simulink model "qsim"  (R2022b)
settings: Solver=VariableStepAuto  StartTime=0.0  StopTime=tmax  MaxStep=dt  RelTol=1e-3
values from neighbouring files (symbols this model uses):
  area = pi*0.42^2    (= 0.554176944093)    [black_brant_vc.m]
  burning_rate = mfuel/burn_time    (= 31.4003701419)    [black_brant_vc.m]
  Cd = [0.386 0.329 0.325 0.469 0.488 0.434 0.389 0.328 0.287 0.255 0.216      0.194 0.184 0.169 0.164 0.154 ]'    [questions.m]
  centrifugal_force = false    [questions.m]
  fthrust = 69.4*10^3    (= 69400)    [black_brant_vc.m]
  G = 6.67430*10^-11    (= 6.6743e-11)    [questions.m]
  M = [0.1 0.5 0.8 1 1.2 1.5 2 2.5 3 3.5 4      4.5 5 5.5 6 6.5]'    [questions.m]
  mfuel = 1018    [black_brant_vc.m]
  mpayload = 100    [black_brant_vc.m]
  mrocket = 243    [black_brant_vc.m]
  nozzle_area = pi*0.34^2    (= 0.363168110755)    [black_brant_vc.m]
  pitch = s*rad    [questions.m]
  v0x = sin(pitch)*v0    [questions.m]
  v0y = sin(pitch)*v0    [questions.m]
  Ve = Isp * G0    [black_brant_vc.m]
  veq = 0    [questions.m]
  x0 = 0    [questions.m]
  y0 = 0    [questions.m]
undefined symbols (not defined in the file or in its folder): D0, H, mearth, P0, r_earth
libraries: simulink x4
settings Model: Creator=mitch  LastModifiedBy=mitch
settings DataIOCC: ReturnWorkspaceOutputs=off

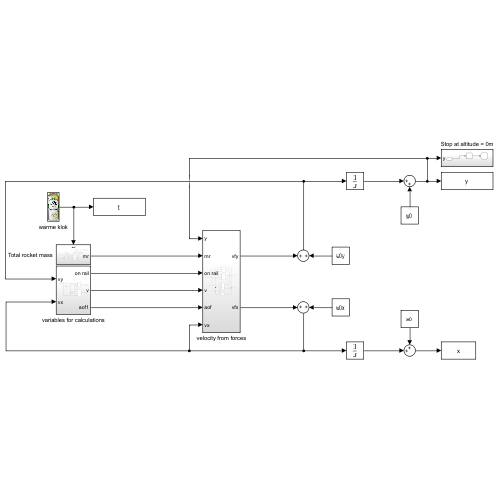
[thumbnail: Simulink's stored preview of the top-level diagram]
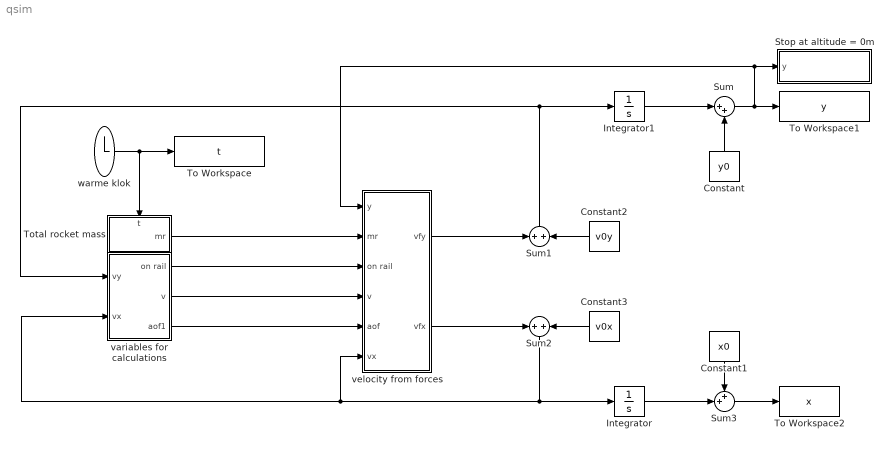
== system qsim ==
  Constant : Constant  Value=y0
  Constant1 : Constant  Value=x0
  Constant2 : Constant  Value=v0y
  Constant3 : Constant  Value=v0x
  Integrator : Integrator
  Integrator1 : Integrator
  Stop at altitude = 0m : Subsystem
  Sum : Sum  Inputs=|++
  Sum1 : Sum
  Sum2 : Sum
  Sum3 : Sum  Inputs=++|
  To Workspace : ToWorkspace  VariableName=t  SampleTime=-1
  To Workspace1 : ToWorkspace  VariableName=y  SampleTime=-1
  To Workspace2 : ToWorkspace  VariableName=x  SampleTime=-1
  Total rocket mass : Subsystem
      settings: PortSchema="{\"entries\":[{\"content\":{\"sides\":[{\"content\":{\"connectorIds\":[]},\"type\":\"ConnectorPlacement.EquallySpacedRectSide\",\"uuid\":\"93486deb-20ea-4256-be89-9e1e72dbb09d\"},{\"content\":{\"connectorIds\":[\"Out1\"],\"side\":\"RIGHT\"},\"type\":\"ConnectorPlacement.EquallySpacedRectSide\",\"uuid\":\"ed0e6263-0b76-41b6-b681-94567fbb2fbf\"},{\"content\":{\"connectorIds\":[\"In1\"],\"side\":\"TOP\"},\"type\":\"ConnectorPlacement.EquallySpacedRectSide\",\"uuid\":\"518b6907-16db-46e5-a33c-d197bc16f302\"}]},\"type\":\"ConnectorPlacement.EquallySpacedConnector\",\"uuid\":\"f80f25e1-82c3-4b04-8094-90952900617d\"}],\"packageUris\":[\"http://schema.mathworks.com/mf0/Connector/R2020b\"],\"version\":\"1.0\"}"
  variables for calculations : Subsystem
  velocity from forces : Subsystem
  warme klok : Clock
      mask Display: image(imread('klok.jpg'))
  wires:
  warme klok/1 -> To Workspace/1, Total rocket mass/1(t)
  Integrator1/1 -> Sum/1
  Sum/1 -> To Workspace1/1, Stop at altitude = 0m/1(y), velocity from forces/1(y)
  Constant/1 -> Sum/2
  Sum1/1 -> Integrator1/1, variables for calculations/1(vy)
  Integrator/1 -> Sum3/2
  Sum3/1 -> To Workspace2/1
  Constant1/1 -> Sum3/1
  Total rocket mass/1(mr) -> velocity from forces/2(mr)
  Sum2/1 -> Integrator/1, variables for calculations/2(vx), velocity from forces/6(vx)
  Constant3/1 -> Sum2/2
  velocity from forces/2(vfx) -> Sum2/1
  variables for calculations/1(on rail) -> velocity from forces/3(on rail)
  variables for calculations/2(v) -> velocity from forces/4(v)
  variables for calculations/3(aof1) -> velocity from forces/5(aof)
  velocity from forces/1(vfy) -> Sum1/1
  Constant2/1 -> Sum1/2

== system qsim/Stop at altitude = 0m ==
  y : Inport
  IsNegative : simulink/Logic and Bit Operations/Compare To Zero  relop=<  OutDataTypeStr=boolean
      settings: LibrarySourceBlock=|
      | simulink/Quick Insert/Logic and Bit
      | Operations/IsNegative
  Stop Simulation : Stop
  wires:
  IsNegative/1 -> Stop Simulation/1
  y/1 -> IsNegative/1

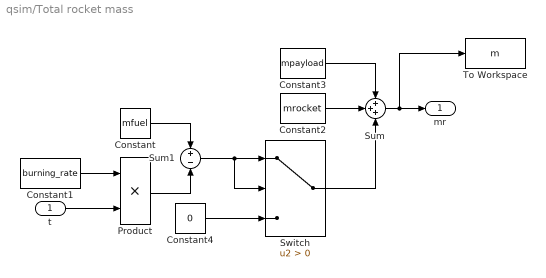
== system qsim/Total rocket mass ==
  t : Inport
  Constant : Constant  Value=mfuel
  Constant1 : Constant  Value=burning_rate
  Constant2 : Constant  Value=mrocket
  Constant3 : Constant  Value=mpayload
  Constant4 : Constant  Value=0
  Product : Product
  Sum : Sum  Inputs=+++
  Sum1 : Sum  Inputs=+-
  Switch : Switch  Criteria=u2 > Threshold  SaturateOnIntegerOverflow=off  InputSameDT=off
  To Workspace : ToWorkspace  VariableName=m  SampleTime=-1
  mr : Outport
  wires:
  Constant3/1 -> Sum/1
  Constant1/1 -> Product/1
  t/1 -> Product/2
  Constant2/1 -> Sum/2
  Constant4/1 -> Switch/3
  Constant/1 -> Sum1/1
  Sum1/1 -> Switch/1, Switch/2
  Product/1 -> Sum1/2
  Switch/1 -> Sum/3
  Sum/1 -> To Workspace/1, mr/1

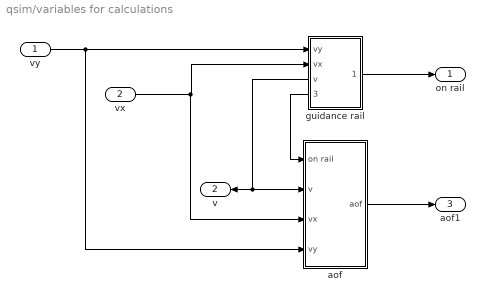
== system qsim/variables for calculations ==
  vy : Inport
  vx : Inport  Port=2
  aof : Subsystem
  guidance rail : Subsystem
      settings: PortSchema="{\"entries\":[{\"content\":{\"sides\":[{\"content\":{\"connectorIds\":[\"In1\",\"In2\",\"Out2\",\"Out3\"]},\"type\":\"ConnectorPlacement.EquallySpacedRectSide\",\"uuid\":\"58d90baa-7253-4a77-a7a7-25666266f078\"},{\"content\":{\"connectorIds\":[\"Out1\"],\"side\":\"RIGHT\"},\"type\":\"ConnectorPlacement.EquallySpacedRectSide\",\"uuid\":\"983a7505-aeb9-4571-80eb-2e5812b070ec\"},{\"content\":{\"connectorIds\":[],\"side\":\"TOP\"},\"type\":\"ConnectorPlacement.EquallySpacedRectSide\",\"uuid\":\"a1f35db6-1c46-42f7-bbcb-98ac4c623d07\"}]},\"type\":\"ConnectorPlacement.EquallySpacedConnector\",\"uuid\":\"73284847-f8fe-421a-b1ed-4d4b0b6e1462\"}],\"packageUris\":[\"http://schema.mathworks.com/mf0/Connector/R2020b\"],\"version\":\"1.0\"}"
  on rail : Outport
  v : Outport  Port=2
  aof1 : Outport  Port=3
  wires:
  guidance rail/3(on rail2) -> aof/1(on rail)
  guidance rail/1(on rail) -> on rail/1
  aof/1(aof) -> aof1/1
  vx/1 -> aof/3(vx), guidance rail/2(vx)
  guidance rail/2(v) -> v/1, aof/2(v)
  vy/1 -> aof/4(vy), guidance rail/1(vy)

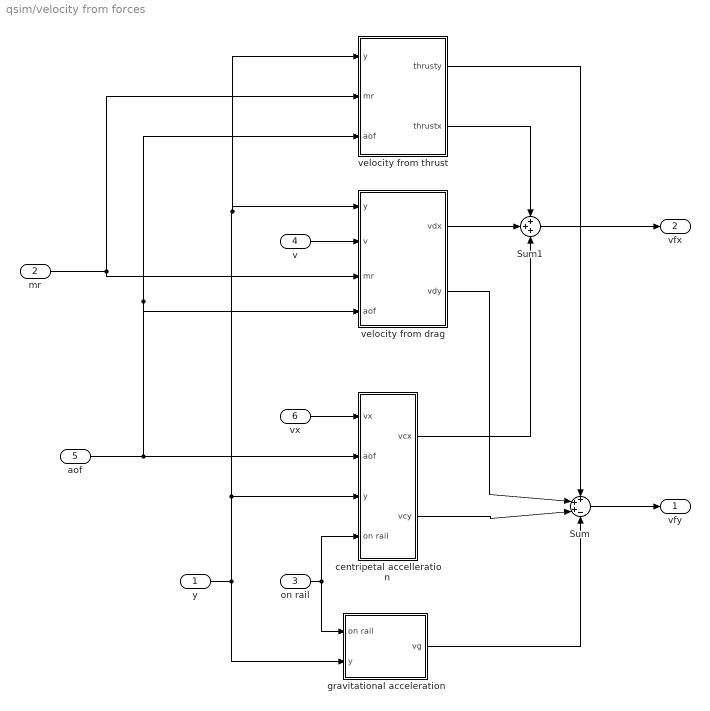
== system qsim/velocity from forces ==
  y : Inport
  mr : Inport  Port=2
  on rail : Inport  Port=3
  v : Inport  Port=4
  aof : Inport  Port=5
  vx : Inport  Port=6
  Sum : Sum  Inputs=+++-
  Sum1 : Sum  Inputs=+++
  centripetal accelleration : Subsystem
  gravitational acceleration : Subsystem
  velocity from drag : Subsystem
  velocity from thrust : Subsystem
  vfy : Outport
  vfx : Outport  Port=2
  wires:
  centripetal accelleration/2(vcy) -> Sum/3
  y/1 -> velocity from thrust/1(y), velocity from drag/1(y), centripetal accelleration/3(y), gravitational acceleration/2(y)
  on rail/1 -> centripetal accelleration/4(on rail), gravitational acceleration/1(on rail)
  mr/1 -> velocity from thrust/2(mr), velocity from drag/3(mr)
  velocity from drag/1(vdx) -> Sum1/2
  v/1 -> velocity from drag/2(v)
  gravitational acceleration/1(vg) -> Sum/4
  vx/1 -> centripetal accelleration/1(vx)
  centripetal accelleration/1(vcx) -> Sum1/3
  velocity from drag/2(vdy) -> Sum/2
  aof/1 -> centripetal accelleration/2(aof), velocity from drag/4(aof), velocity from thrust/3(aof)
  velocity from thrust/2(thrustx) -> Sum1/1
  velocity from thrust/1(thrusty) -> Sum/1
  Sum1/1 -> vfx/1
  Sum/1 -> vfy/1

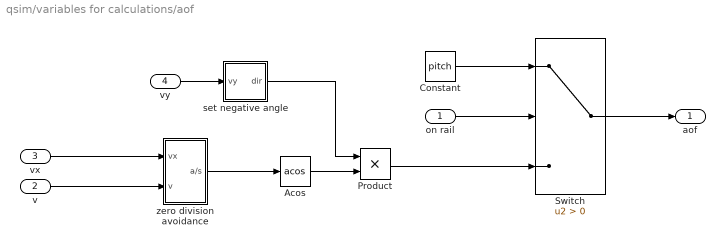
== system qsim/variables for calculations/aof ==
  on rail : Inport
  v : Inport  Port=2
  vx : Inport  Port=3
  vy : Inport  Port=4
  Acos : Trigonometry  Operator=acos
  Constant : Constant  Value=pitch
  Product : Product
  Switch : Switch  Criteria=u2 > Threshold  SaturateOnIntegerOverflow=off  InputSameDT=off
  set negative angle : Subsystem
  zero division avoidance : Subsystem
  aof : Outport
  wires:
  Switch/1 -> aof/1
  Constant/1 -> Switch/1
  on rail/1 -> Switch/2
  vx/1 -> zero division avoidance/1(vx)
  v/1 -> zero division avoidance/2(v)
  zero division avoidance/1(a/s) -> Acos/1
  Acos/1 -> Product/2
  Product/1 -> Switch/3
  vy/1 -> set negative angle/1(vy)
  set negative angle/1(dir) -> Product/1

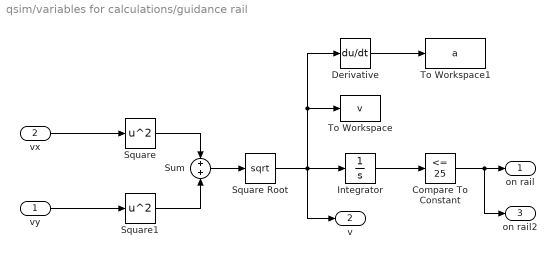
== system qsim/variables for calculations/guidance rail ==
  vy : Inport
  vx : Inport  Port=2
  Compare To Constant : simulink/Logic and Bit Operations/Compare To Constant  relop=<=  const=25  OutDataTypeStr=boolean
  Derivative : Derivative
  Integrator : Integrator
  Square : Math  Operator=square
  Square Root : Sqrt
  Square1 : Math  Operator=square
  Sum : Sum
  To Workspace : ToWorkspace  VariableName=v  SampleTime=-1
  To Workspace1 : ToWorkspace  VariableName=a  SampleTime=-1
  on rail : Outport
  v : Outport  Port=2
  on rail2 : Outport  Port=3
  wires:
  vy/1 -> Square1/1
  Square1/1 -> Sum/2
  Square/1 -> Sum/1
  Sum/1 -> Square Root/1
  Square Root/1 -> v/1, Derivative/1, To Workspace/1, Integrator/1
  Integrator/1 -> Compare To Constant/1
  Compare To Constant/1 -> on rail2/1, on rail/1
  vx/1 -> Square/1
  Derivative/1 -> To Workspace1/1

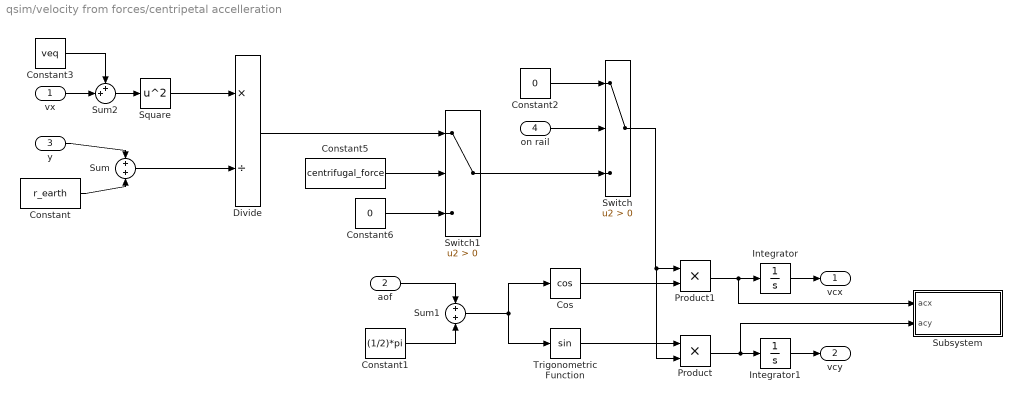
== system qsim/velocity from forces/centripetal accelleration ==
  vx : Inport
  aof : Inport  Port=2
  y : Inport  Port=3
  on rail : Inport  Port=4
  Constant : Constant  Value=r_earth
  Constant1 : Constant  Value=(1/2)*pi
  Constant2 : Constant  Value=0
  Constant3 : Constant  Value=veq
  Constant5 : Constant  Value=centrifugal_force
  Constant6 : Constant  Value=0
  Cos : Trigonometry  Operator=cos
  Divide : Product  Inputs=*/
  Integrator : Integrator
  Integrator1 : Integrator
  Product : Product
  Product1 : Product
  Square : Math  Operator=square
  Subsystem : Subsystem
  Sum : Sum
  Sum1 : Sum
  Sum2 : Sum  Inputs=++|
  Switch : Switch  Criteria=u2 > Threshold  SaturateOnIntegerOverflow=off  InputSameDT=off
  Switch1 : Switch  Criteria=u2 > Threshold  SaturateOnIntegerOverflow=off  InputSameDT=off
  Trigonometric Function : Trigonometry
  vcx : Outport
  vcy : Outport  Port=2
  wires:
  Constant/1 -> Sum/2
  y/1 -> Sum/1
  Square/1 -> Divide/1
  Sum/1 -> Divide/2
  aof/1 -> Sum1/1
  Constant1/1 -> Sum1/2
  Sum1/1 -> Trigonometric Function/1, Cos/1
  Cos/1 -> Product1/2
  Trigonometric Function/1 -> Product/1
  Integrator/1 -> vcx/1
  Product1/1 -> Subsystem/1(acx), Integrator/1
  Integrator1/1 -> vcy/1
  Product/1 -> Subsystem/2(acy), Integrator1/1
  Constant5/1 -> Switch1/2
  Constant6/1 -> Switch1/3
  Divide/1 -> Switch1/1
  on rail/1 -> Switch/2
  Constant2/1 -> Switch/1
  Switch1/1 -> Switch/3
  Switch/1 -> Product/2, Product1/1
  Sum2/1 -> Square/1
  vx/1 -> Sum2/2
  Constant3/1 -> Sum2/1

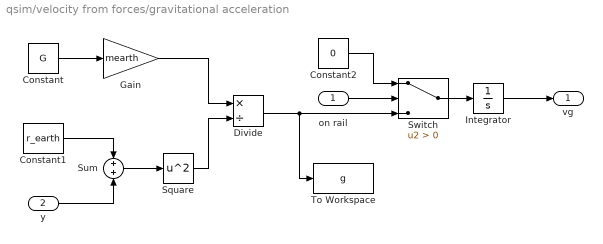
== system qsim/velocity from forces/gravitational acceleration ==
  on rail : Inport
  y : Inport  Port=2
  Constant : Constant  Value=G
  Constant1 : Constant  Value=r_earth
  Constant2 : Constant  Value=0
  Divide : Product  Inputs=*/
  Gain : Gain  Gain=mearth
  Integrator : Integrator
  Square : Math  Operator=square
  Sum : Sum
  Switch : Switch  Criteria=u2 > Threshold  SaturateOnIntegerOverflow=off  InputSameDT=off
  To Workspace : ToWorkspace  VariableName=g  SampleTime=-1
  vg : Outport
  wires:
  y/1 -> Sum/2
  Constant1/1 -> Sum/1
  Constant/1 -> Gain/1
  Gain/1 -> Divide/1
  Sum/1 -> Square/1
  Square/1 -> Divide/2
  Divide/1 -> Switch/3, To Workspace/1
  on rail/1 -> Switch/2
  Switch/1 -> Integrator/1
  Integrator/1 -> vg/1
  Constant2/1 -> Switch/1

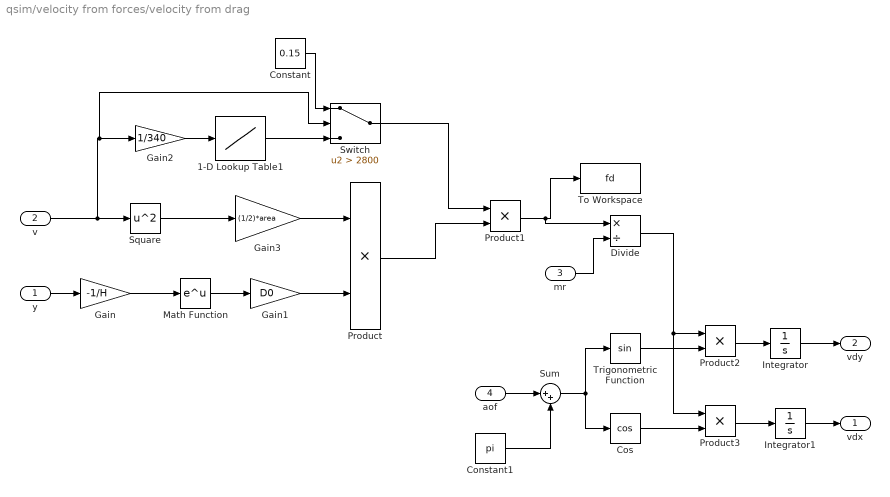
== system qsim/velocity from forces/velocity from drag ==
  y : Inport
  v : Inport  Port=2
  mr : Inport  Port=3
  aof : Inport  Port=4
  1-D Lookup Table1 : Lookup_n-D  NumberOfTableDimensions=1  BreakpointsForDimension1=M  Table=Cd  InternalRulePriority=Speed  RndMeth=Simplest
  Constant : Constant  Value=0.15
  Constant1 : Constant  Value=pi
  Cos : Trigonometry  Operator=cos
  Divide : Product  Inputs=*/
  Gain : Gain  Gain=-1/H
  Gain1 : Gain  Gain=D0
  Gain2 : Gain  Gain=1/340
  Gain3 : Gain  Gain=(1/2)*area
  Integrator : Integrator
  Integrator1 : Integrator
  Math Function : Math
  Product{,1..3} (4 alike) : Product
  Square : Math  Operator=square
  Sum : Sum  Inputs=|++
  Switch : Switch  Criteria=u2 > Threshold  Threshold=2800  SaturateOnIntegerOverflow=off  InputSameDT=off
  To Workspace : ToWorkspace  VariableName=fd  SampleTime=-1
  Trigonometric Function : Trigonometry
  vdx : Outport
  vdy : Outport  Port=2
  wires:
  y/1 -> Gain/1
  Gain/1 -> Math Function/1
  Math Function/1 -> Gain1/1
  Gain1/1 -> Product/2
  Square/1 -> Gain3/1
  Gain3/1 -> Product/1
  Constant/1 -> Switch/1
  1-D Lookup Table1/1 -> Switch/3
  Gain2/1 -> 1-D Lookup Table1/1
  v/1 -> Switch/2, Gain2/1, Square/1
  Switch/1 -> Product1/1
  Product/1 -> Product1/2
  Product1/1 -> Divide/1, To Workspace/1
  mr/1 -> Divide/2
  aof/1 -> Sum/1
  Constant1/1 -> Sum/2
  Sum/1 -> Cos/1, Trigonometric Function/1
  Cos/1 -> Product3/2
  Trigonometric Function/1 -> Product2/2
  Divide/1 -> Product3/1, Product2/1
  Product2/1 -> Integrator/1
  Integrator/1 -> vdy/1
  Integrator1/1 -> vdx/1
  Product3/1 -> Integrator1/1

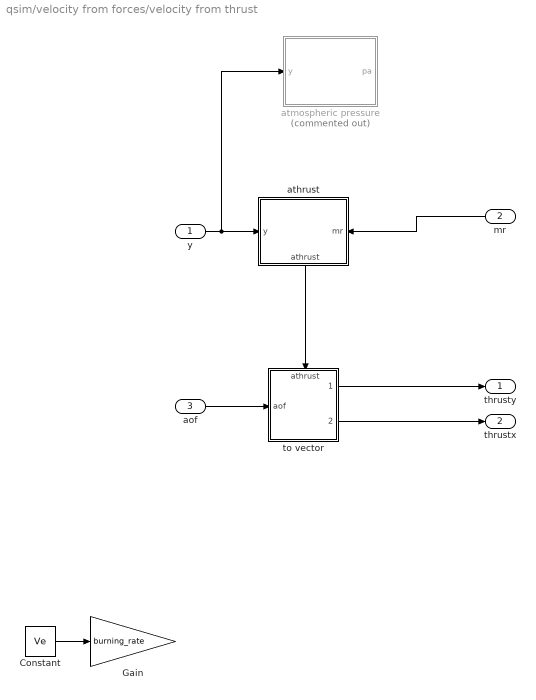
== system qsim/velocity from forces/velocity from thrust ==
  y : Inport
  mr : Inport  Port=2
  aof : Inport  Port=3
  Constant : Constant  Value=Ve
  Gain : Gain  Gain=burning_rate
  athrust : Subsystem
      settings: PortSchema="{\"entries\":[{\"content\":{\"sides\":[{\"content\":{\"connectorIds\":[\"In1\"]},\"type\":\"ConnectorPlacement.EquallySpacedRectSide\",\"uuid\":\"38b57bf2-f272-494c-b87c-d8faf890034d\"},{\"content\":{\"connectorIds\":[\"In2\"],\"side\":\"RIGHT\"},\"type\":\"ConnectorPlacement.EquallySpacedRectSide\",\"uuid\":\"28bf3ef2-f049-46a8-a4c1-ef06de2542f6\"},{\"content\":{\"connectorIds\":[],\"side\":\"TOP\"},\"type\":\"ConnectorPlacement.EquallySpacedRectSide\",\"uuid\":\"9b9cc41a-51fa-40c5-9d78-95f4222731b9\"},{\"content\":{\"connectorIds\":[\"Out1\"],\"side\":\"BOTTOM\"},\"type\":\"ConnectorPlacement.EquallySpacedRectSide\",\"uuid\":\"8c2dcb6d-3fb6-40dd-9d2b-9aea55817220\"}]},\"type\":\"ConnectorPlacement.EquallySpacedConnector\",\"uuid\":\"881def1f-c4e6-4073-9099-93e1a9067931\"}],\"packageUris\":[\"http://schema.mathworks.com/mf0/Connector/R2020b\"],\"version\":\"1.0\"}"
  atmospheric pressure : Subsystem  Commented=on
  to vector : Subsystem
      settings: PortSchema="{\"entries\":[{\"content\":{\"sides\":[{\"content\":{\"connectorIds\":[\"In1\"]},\"type\":\"ConnectorPlacement.EquallySpacedRectSide\",\"uuid\":\"eef117ae-5443-4bd2-924b-a9bef27ce47b\"},{\"content\":{\"connectorIds\":[\"Out1\",\"Out2\"],\"side\":\"RIGHT\"},\"type\":\"ConnectorPlacement.EquallySpacedRectSide\",\"uuid\":\"5f20767f-5b49-4661-976c-87d1d852a688\"},{\"content\":{\"connectorIds\":[\"In2\"],\"side\":\"TOP\"},\"type\":\"ConnectorPlacement.EquallySpacedRectSide\",\"uuid\":\"987dd712-ddbe-4dae-902f-65e809d67914\"}]},\"type\":\"ConnectorPlacement.EquallySpacedConnector\",\"uuid\":\"11712861-a8e2-4e00-8f3c-6518121a0119\"}],\"packageUris\":[\"http://schema.mathworks.com/mf0/Connector/R2020b\"],\"version\":\"1.0\"}"
  thrusty : Outport
  thrustx : Outport  Port=2
  wires:
  aof/1 -> to vector/1(aof)
  mr/1 -> athrust/2(mr)
  athrust/1(athrust) -> to vector/2(athrust)
  to vector/1(thrusty) -> thrusty/1
  to vector/2(thrustx) -> thrustx/1
  y/1 -> atmospheric pressure/1(y), athrust/1(y)
  Constant/1 -> Gain/1

== system qsim/variables for calculations/aof/set negative angle ==
  vy : Inport
  Abs : Abs  SaturateOnIntegerOverflow=off
  zero division avoidance 2 : Subsystem
  dir : Outport
  wires:
  Abs/1 -> zero division avoidance 2/2(|vy|)
  vy/1 -> zero division avoidance 2/1(vy), Abs/1
  zero division avoidance 2/1(dir) -> dir/1

== system qsim/variables for calculations/aof/zero division avoidance ==
  vx : Inport
  v : Inport  Port=2
  Compare To Zero : simulink/Logic and Bit Operations/Compare To Zero  relop===  OutDataTypeStr=boolean
  Divide : Product  Inputs=*/
  Switch : Switch  Criteria=u2 > Threshold  SaturateOnIntegerOverflow=off  InputSameDT=off
  a/s : Outport
  wires:
  vx/1 -> Switch/1, Divide/1
  Divide/1 -> a/s/1
  Compare To Zero/1 -> Switch/2
  Switch/1 -> Divide/2
  v/1 -> Switch/3, Compare To Zero/1

== system qsim/velocity from forces/centripetal accelleration/Subsystem ==
  acx : Inport
  acy : Inport  Port=2
  Sqrt : Sqrt
  Square1 : Math  Operator=square
  Square2 : Math  Operator=square
  Sum2 : Sum
  To Workspace : ToWorkspace  VariableName=ac  SampleTime=-1
  wires:
  Square1/1 -> Sum2/1
  acx/1 -> Square1/1
  Square2/1 -> Sum2/2
  Sqrt/1 -> To Workspace/1
  acy/1 -> Square2/1
  Sum2/1 -> Sqrt/1

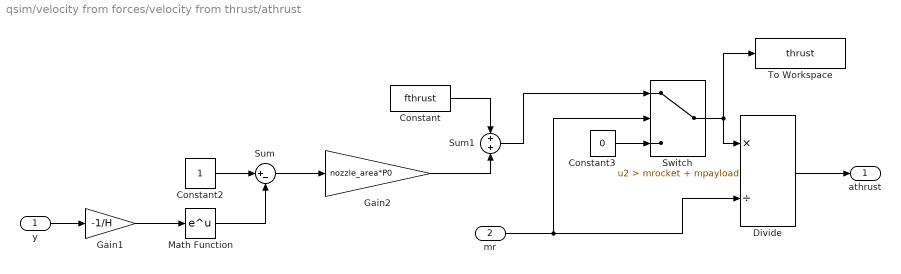
== system qsim/velocity from forces/velocity from thrust/athrust ==
  y : Inport
  mr : Inport  Port=2
  Constant : Constant  Value=fthrust
  Constant2 : Constant
  Constant3 : Constant  Value=0
  Divide : Product  Inputs=*/
  Gain1 : Gain  Gain=-1/H
  Gain2 : Gain  Gain=nozzle_area*P0
  Math Function : Math
  Sum : Sum  Inputs=|+-
  Sum1 : Sum
  Switch : Switch  Criteria=u2 > Threshold  Threshold=mrocket + mpayload  SaturateOnIntegerOverflow=off  InputSameDT=off
  To Workspace : ToWorkspace  VariableName=thrust  SampleTime=-1
  athrust : Outport
  wires:
  Math Function/1 -> Sum/2
  Gain1/1 -> Math Function/1
  Constant2/1 -> Sum/1
  y/1 -> Gain1/1
  Gain2/1 -> Sum1/2
  Constant/1 -> Sum1/1
  mr/1 -> Divide/2, Switch/2
  Constant3/1 -> Switch/3
  Divide/1 -> athrust/1
  Switch/1 -> Divide/1, To Workspace/1
  Sum1/1 -> Switch/1
  Sum/1 -> Gain2/1

== system qsim/velocity from forces/velocity from thrust/atmospheric pressure ==
  y : Inport
  Constant2 : Constant  Value=H
  Divide : Product  Inputs=*/
  Gain1 : Gain  Gain=-1
  Gain2 : Gain  Gain=P0
  Math Function : Math
  pa : Outport
  wires:
  Gain1/1 -> Divide/1
  Math Function/1 -> Gain2/1
  Constant2/1 -> Divide/2
  Gain2/1 -> pa/1
  Divide/1 -> Math Function/1
  y/1 -> Gain1/1

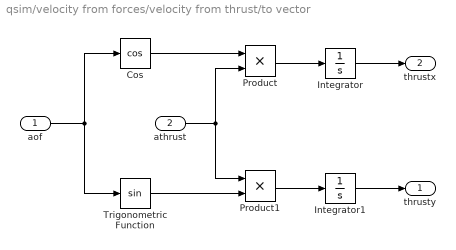
== system qsim/velocity from forces/velocity from thrust/to vector ==
  aof : Inport
  athrust : Inport  Port=2
  Cos : Trigonometry  Operator=cos
  Integrator : Integrator
  Integrator1 : Integrator
  Product : Product
  Product1 : Product
  Trigonometric Function : Trigonometry
  thrusty : Outport
  thrustx : Outport  Port=2
  wires:
  Cos/1 -> Product/1
  Trigonometric Function/1 -> Product1/2
  aof/1 -> Trigonometric Function/1, Cos/1
  athrust/1 -> Product1/1, Product/2
  Product/1 -> Integrator/1
  Integrator/1 -> thrustx/1
  Product1/1 -> Integrator1/1
  Integrator1/1 -> thrusty/1

== system qsim/variables for calculations/aof/set negative angle/zero division avoidance 2 ==
  vy : Inport
  |vy| : Inport  Port=2
  Compare To Zero : simulink/Logic and Bit Operations/Compare To Zero  relop===  OutDataTypeStr=boolean
  Constant : Constant
  Divide : Product  Inputs=*/
  Switch : Switch  Criteria=u2 > Threshold  SaturateOnIntegerOverflow=off  InputSameDT=off
  dir : Outport
  wires:
  vy/1 -> Divide/1
  Divide/1 -> dir/1
  Compare To Zero/1 -> Switch/2
  Switch/1 -> Divide/2
  |vy|/1 -> Switch/3, Compare To Zero/1
  Constant/1 -> Switch/1
